simulink model "bh_model_crank_dynamics_b_version"  (R2022a)
settings: Solver=ode15s  StartTime=0.0  StopTime=45  RelTol=1e-8  AbsTol=1e-8  EnableMultiTasking=on
undefined symbols (not defined in the file): IC, params, sigbuilder_block, X, Y, Z
libraries: simulink_extras x27, sm_lib x21, nesl_utility x19, simulink x2
(part 2 of 2)

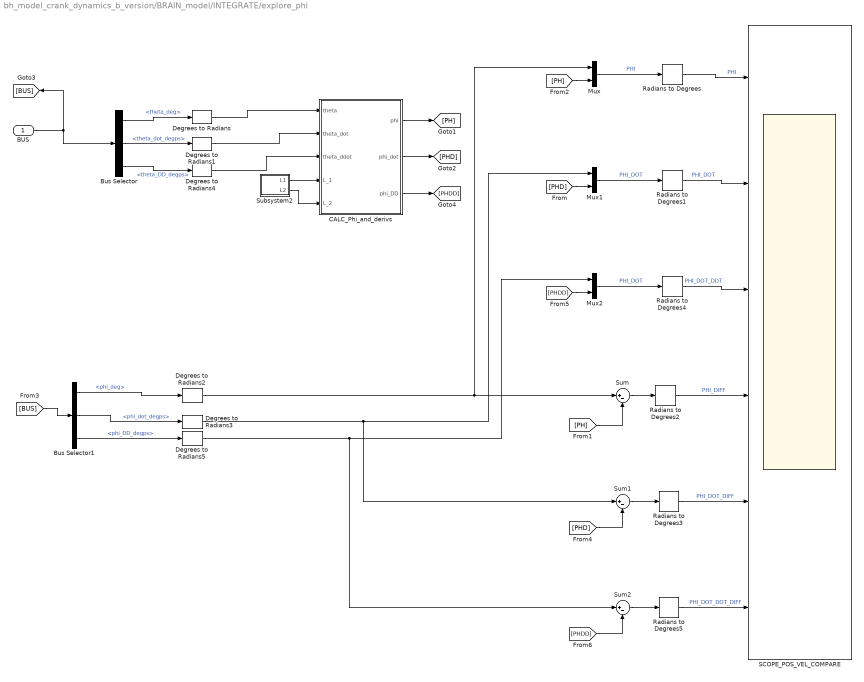
== system bh_model_crank_dynamics_b_version/BRAIN_model/INTEGRATE/explore_phi ==
  BUS : Inport
  Bus Selector : BusSelector  OutputSignals=theta_deg,theta_dot_degps,theta_DD_degps
  Bus Selector1 : BusSelector  OutputSignals=phi_deg,phi_dot_degps,phi_DD_degps
  CALC_Phi_and_derivs : MATLAB Function  TreatAsAtomicUnit=on
  Degrees to Radians{,1..5} (6 alike) : simulink_extras/Transformations/Degrees to Radians
  Mux : Mux  Inputs=2
  Mux1 : Mux  Inputs=2
  Mux2 : Mux  Inputs=2
  Radians to Degrees{,1..5} (6 alike) : simulink_extras/Transformations/Radians to Degrees
  SCOPE_POS_VEL_COMPARE : Scope  NumInputPorts=6
  Subsystem2 : Subsystem
  Sum : Sum  Inputs=|+-
  Sum1 : Sum  Inputs=|+-
  Sum2 : Sum  Inputs=|+-
  wires:
  Subsystem2/1(L1) -> CALC_Phi_and_derivs/4(L_1)
  Subsystem2/2(L2) -> CALC_Phi_and_derivs/5(L_2)
  BUS/1 -> [BUS], Bus Selector/1
  Degrees to Radians/1 -> CALC_Phi_and_derivs/1(theta)
  Degrees to Radians1/1 -> CALC_Phi_and_derivs/2(theta_dot)
  Radians to Degrees/1 -> SCOPE_POS_VEL_COMPARE/1  "PHI"
  Radians to Degrees1/1 -> SCOPE_POS_VEL_COMPARE/2  "PHI_DOT"
  CALC_Phi_and_derivs/2(phi_dot) -> [PHD]
  CALC_Phi_and_derivs/1(phi) -> [PH]
  [PH] -> Mux/2
  [PHD] -> Mux1/2
  [BUS] -> Bus Selector1/1
  Bus Selector1/2 -> Degrees to Radians3/1  "<phi_dot_degps>"
  Bus Selector1/1 -> Degrees to Radians2/1  "<phi_deg>"
  Degrees to Radians2/1 -> Mux/1, Sum/1
  [PH] -> Sum/2
  [PHD] -> Sum1/2
  Degrees to Radians3/1 -> Sum1/1, Mux1/1
  Sum1/1 -> Radians to Degrees3/1
  Sum/1 -> Radians to Degrees2/1
  Mux/1 -> Radians to Degrees/1  "PHI"
  Mux1/1 -> Radians to Degrees1/1  "PHI_DOT"
  Degrees to Radians4/1 -> CALC_Phi_and_derivs/3(theta_ddot)
  Bus Selector/1 -> Degrees to Radians/1  "<theta_deg>"
  Bus Selector/2 -> Degrees to Radians1/1  "<theta_dot_degps>"
  Bus Selector/3 -> Degrees to Radians4/1  "<theta_DD_degps>"
  CALC_Phi_and_derivs/3(phi_DD) -> [PHDD]
  Bus Selector1/3 -> Degrees to Radians5/1  "<phi_DD_degps>"
  Radians to Degrees3/1 -> SCOPE_POS_VEL_COMPARE/5  "PHI_DOT_DIFF"
  Radians to Degrees2/1 -> SCOPE_POS_VEL_COMPARE/4  "PHI_DIFF"
  Mux2/1 -> Radians to Degrees4/1  "PHI_DOT"
  [PHDD] -> Mux2/2
  Radians to Degrees4/1 -> SCOPE_POS_VEL_COMPARE/3  "PHI_DOT_DOT"
  Degrees to Radians5/1 -> Sum2/1, Mux2/1
  Radians to Degrees5/1 -> SCOPE_POS_VEL_COMPARE/6  "PHI_DOT_DOT_DIFF"
  [PHDD] -> Sum2/2
  Sum2/1 -> Radians to Degrees5/1

== system bh_model_crank_dynamics_b_version/SIMSCAPE_MODEL/Subsystem1/Subsystem ==
  ANG : Inport
  AXIS : Inport  Port=2
  Compare To Zero : simulink/Logic and Bit Operations/Compare To Zero  relop=>=  OutDataTypeStr=boolean
  Gain : Gain  Gain=-1
  Selector : Selector  InputPortWidth=3  IndexOptions=Index vector (dialog)  Indices=3  OutputSizes=1
  Switch : Switch  Criteria=u2 > Threshold  SaturateOnIntegerOverflow=off  InputSameDT=off
  ANG_OUT : Outport
  wires:
  AXIS/1 -> Selector/1
  Selector/1 -> Compare To Zero/1
  Switch/1 -> ANG_OUT/1
  ANG/1 -> Gain/1, Switch/1
  Compare To Zero/1 -> Switch/2
  Gain/1 -> Switch/3

== system bh_model_crank_dynamics_b_version/SIMSCAPE_MODEL/Subsystem2/Subsystem ==
  ANG : Inport
  AXIS : Inport  Port=2
  Compare To Zero : simulink/Logic and Bit Operations/Compare To Zero  relop=>=  OutDataTypeStr=boolean
  Gain : Gain  Gain=-1
  Selector : Selector  InputPortWidth=3  IndexOptions=Index vector (dialog)  Indices=3  OutputSizes=1
  Switch : Switch  Criteria=u2 > Threshold  SaturateOnIntegerOverflow=off  InputSameDT=off
  ANG_OUT : Outport
  wires:
  AXIS/1 -> Selector/1
  Selector/1 -> Compare To Zero/1
  Switch/1 -> ANG_OUT/1
  ANG/1 -> Gain/1, Switch/1
  Compare To Zero/1 -> Switch/2
  Gain/1 -> Switch/3

== system bh_model_crank_dynamics_b_version/SIMSCAPE_MODEL/make_BUS/pm_pi ==
  rad_in : Inport
  Trigonometric Function : Trigonometry  Operator=atan2
  Trigonometric Function1 : Trigonometry
  Trigonometric Function2 : Trigonometry  Operator=cos
  rad_out : Outport
  wires:
  rad_in/1 -> Trigonometric Function2/1, Trigonometric Function1/1
  Trigonometric Function2/1 -> Trigonometric Function/2
  Trigonometric Function1/1 -> Trigonometric Function/1
  Trigonometric Function/1 -> rad_out/1

== system bh_model_crank_dynamics_b_version/SIMSCAPE_MODEL/make_BUS/pm_pi1 ==
  rad_in : Inport
  Trigonometric Function : Trigonometry  Operator=atan2
  Trigonometric Function1 : Trigonometry
  Trigonometric Function2 : Trigonometry  Operator=cos
  rad_out : Outport
  wires:
  rad_in/1 -> Trigonometric Function2/1, Trigonometric Function1/1
  Trigonometric Function2/1 -> Trigonometric Function/2
  Trigonometric Function1/1 -> Trigonometric Function/1
  Trigonometric Function/1 -> rad_out/1

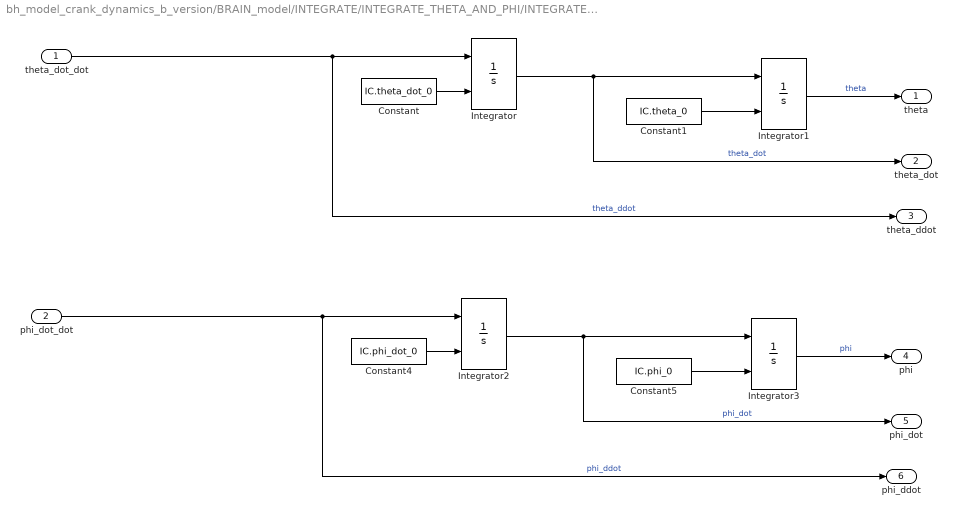
== system bh_model_crank_dynamics_b_version/BRAIN_model/INTEGRATE/INTEGRATE_THETA_AND_PHI/INTEGRATE_SYS ==
  theta_dot_dot : Inport
  phi_dot_dot : Inport  Port=2
  Constant : Constant  Value=IC.theta_dot_0
  Constant1 : Constant  Value=IC.theta_0
  Constant4 : Constant  Value=IC.phi_dot_0
  Constant5 : Constant  Value=IC.phi_0
  Integrator : Integrator  InitialConditionSource=external
  Integrator1 : Integrator  InitialConditionSource=external  WrapState=on
  Integrator2 : Integrator  InitialConditionSource=external
  Integrator3 : Integrator  InitialConditionSource=external  WrapState=on
  theta : Outport
  theta_dot : Outport  Port=2
  theta_ddot : Outport  Port=3
  phi : Outport  Port=4
  phi_dot : Outport  Port=5
  phi_ddot : Outport  Port=6
  wires:
  Integrator1/1 -> theta/1  "theta"
  theta_dot_dot/1 -> Integrator/1, theta_ddot/1  "theta_ddot"
  Constant/1 -> Integrator/2
  Integrator/1 -> theta_dot/1, Integrator1/1  "theta_dot"
  Constant1/1 -> Integrator1/2
  Constant5/1 -> Integrator3/2
  Integrator2/1 -> phi_dot/1, Integrator3/1  "phi_dot"
  phi_dot_dot/1 -> Integrator2/1, phi_ddot/1  "phi_ddot"
  Integrator3/1 -> phi/1  "phi"
  Constant4/1 -> Integrator2/2

== system bh_model_crank_dynamics_b_version/BRAIN_model/INTEGRATE/Make_BUS/pm_pi ==
  rad_in : Inport
  Trigonometric Function : Trigonometry  Operator=atan2
  Trigonometric Function1 : Trigonometry
  Trigonometric Function2 : Trigonometry  Operator=cos
  rad_out : Outport
  wires:
  rad_in/1 -> Trigonometric Function2/1, Trigonometric Function1/1
  Trigonometric Function2/1 -> Trigonometric Function/2
  Trigonometric Function1/1 -> Trigonometric Function/1
  Trigonometric Function/1 -> rad_out/1

== system bh_model_crank_dynamics_b_version/BRAIN_model/INTEGRATE/Make_BUS/pm_pi1 ==
  rad_in : Inport
  Trigonometric Function : Trigonometry  Operator=atan2
  Trigonometric Function1 : Trigonometry
  Trigonometric Function2 : Trigonometry  Operator=cos
  rad_out : Outport
  wires:
  rad_in/1 -> Trigonometric Function2/1, Trigonometric Function1/1
  Trigonometric Function2/1 -> Trigonometric Function/2
  Trigonometric Function1/1 -> Trigonometric Function/1
  Trigonometric Function/1 -> rad_out/1

== system bh_model_crank_dynamics_b_version/BRAIN_model/INTEGRATE/explore_phi/Subsystem2 ==
  Constant4 : Constant  Value=params.L_1
  Constant5 : Constant  Value=params.L_2
  L1 : Outport
  L2 : Outport  Port=2
  wires:
  Constant5/1 -> L2/1
  Constant4/1 -> L1/1

== matlab function bh_model_crank_dynamics_b_version/BRAIN_model/my_EOM1 ==
  data: F_P input; A output; I_A1 input; I_G2 input; L_1 input; L_2 input; b_A input; b_P input; g input; m_1 input; m_2 input; m_P input; phi input; phi_dot input; tau_A input; theta input; theta_dot input; b output
function [A,b] = my_EOM(F_P,I_A1,I_G2,L_1,L_2,b_A,b_P,g,m_1,m_2,m_P,phi,phi_dot,tau_A,theta,theta_dot)
%#codegen

%    This function was generated by the Symbolic Math Toolbox version 9.1.
%    26-Jun-2022 15:53:52

t2 = cos(phi);
t3 = cos(theta);
t4 = sin(phi);
t5 = sin(theta);
t6 = phi_dot.^2;
t7 = theta_dot.^2;
t8 = L_1.*t3;
t10 = L_1.*t5.*t7;
t11 = (L_2.*t2)./2.0;
t12 = (L_2.*t4)./2.0;
A = reshape([L_1.*m_1.*t5.*(-1.0./2.0),(m_1.*t8)./2.0,I_A1,-L_1.*m_2.*t5,m_2.*t8,0.0,-L_1.*m_P.*t5,0.0,t8,0.0,0.0,0.0,L_2.*m_2.*t4.*(-1.0./2.0),L_2.*m_2.*t2.*(-1.0./2.0),-I_G2,-L_2.*m_P.*t4,0.0,-L_2.*t2,-1.0,0.0,0.0,0.0,0.0,0.0,0.0,0.0,0.0,0.0,-1.0,0.0,0.0,0.0,0.0,0.0,0.0,0.0,1.0,0.0,-L_1.*t5,-1.0,0.0,t12,0.0,0.0,0.0,0.0,1.0,t8,0.0,-1.0,t11,0.0,0.0,0.0,0.0,0.0,0.0,1.0,0.0,t12,-1.0,0.0,0.0,0.0,0.0,0.0,0.0,1.0,t11,0.0,-1.0,0.0,0.0,0.0,0.0,0.0,0.0,0.0,0.0,-1.0,0.0],[9,9]);
if nargout > 1
    t9 = t7.*t8;
    b = [(m_1.*t9)./2.0;-g.*m_1+(m_1.*t10)./2.0;tau_A-b_A.*theta_dot-(g.*m_1.*t8)./2.0;m_2.*(t9+t6.*t11);-g.*m_2+m_2.*(t10-(L_2.*t4.*t6)./2.0);0.0;F_P+m_P.*(t9+L_2.*t2.*t6)+b_P.*(L_2.*phi_dot.*t4+L_1.*t5.*theta_dot);-g.*m_P;t10-L_2.*t4.*t6];
end

== matlab function bh_model_crank_dynamics_b_version/SIMSCAPE_MODEL/make_R_BUS/Convert_BODY_fixed to WORLD ==
  data: xy_B_vec input size=2; xy_W_vec output size=[2,1]; gamma input size=1
function xy_W_vec = fcn(xy_B_vec, gamma)

    gRb      = [  cos(gamma),  -sin(gamma);
                  sin(gamma),   cos(gamma)   ];
      
    xy_W_vec = gRb * xy_B_vec(:);

end

== matlab function bh_model_crank_dynamics_b_version/BRAIN_model/INTEGRATE/CALC_P_pos_and_vel ==
  data: L_1 input; x_P output; L_2 input; theta input; theta_dot input; theta_ddot input; phi input; phi_dot input; v_P output; a_P output; phi_ddot input
function [x_P, v_P, a_P] = fcn(L_1, L_2, theta, theta_dot, theta_ddot, phi, phi_dot, phi_ddot)

    x_P =    L_1*cos(theta)  +  L_2*cos(phi);
    
    v_P =   -L_1*sin(theta)*theta_dot  - L_2*sin(phi)*phi_dot;  % need this for the damping Force
    
    a_P =   (-L_1*cos(theta)*theta_dot^2   + -L_1*sin(theta)*theta_ddot)   +   ...
            (-L_2*cos(phi)*phi_dot^2       + -L_2*sin(phi)*phi_ddot);

end

== matlab function bh_model_crank_dynamics_b_version/BRAIN_model/INTEGRATE/explore_phi/CALC_Phi_and_derivs ==
  data: theta input size=1; theta_dot input size=1; theta_ddot input; L_1 input size=1; phi output double size=1; L_2 input size=1; phi_dot output double size=1; phi_DD output
function [phi, phi_dot, phi_DD ] = fcn(theta,theta_dot,theta_ddot, L_1, L_2)

 phi      = asin(  (L_1/L_2) * sin(theta)  );

 phi_dot  = L_1*cos(theta)*theta_dot/(L_2*cos(phi));

% 
% EQ_9 = (-L_1*sin(theta)*(theta_dot^2) + L_1*cos(theta)*theta_ddot) == ...
%        (-L_2*sin(phi)*(phi_dot^2)     + L_2*cos(phi)*phi_ddot);


 phi_DD   = (-L_1*sin(theta)*(theta_dot^2) + L_1*cos(theta)*theta_ddot  + ...
             L_2*sin(phi)*(phi_dot^2) )/(L_2*cos(phi));


end
